simulink model "SSR_IFFT"  (R2020a)
settings: Solver=VariableStepAuto  StartTime=0.0  StopTime=2E-9*N/SSR*8  RelTol=1e-3
PreLoadFcn:
  | N=1024;
  | SSR=4;
undefined symbols (not defined in the file): Low
libraries: xbsIndex_r4 x10, xrbsSSR_Library x5, dspbuff3 x1, xbsCopyrightNotice_r4 x1, dspxfrm3 x1, dspswit3 x1
settings Model: Creator=admin  LastModifiedBy=viswanad
settings DataIOCC: ReturnWorkspaceOutputs=off
settings DebuggingCC: ArithmeticOperatorsInVariantConditions=warning
settings SFSimCC: SimUseLocalCustomCode=off  CustomCodeUndefinedFunction=UseInterfaceOnly
settings RTWCC: RTWUseLocalCustomCode=off
settings CodeAppCC: StateflowObjectComments=on

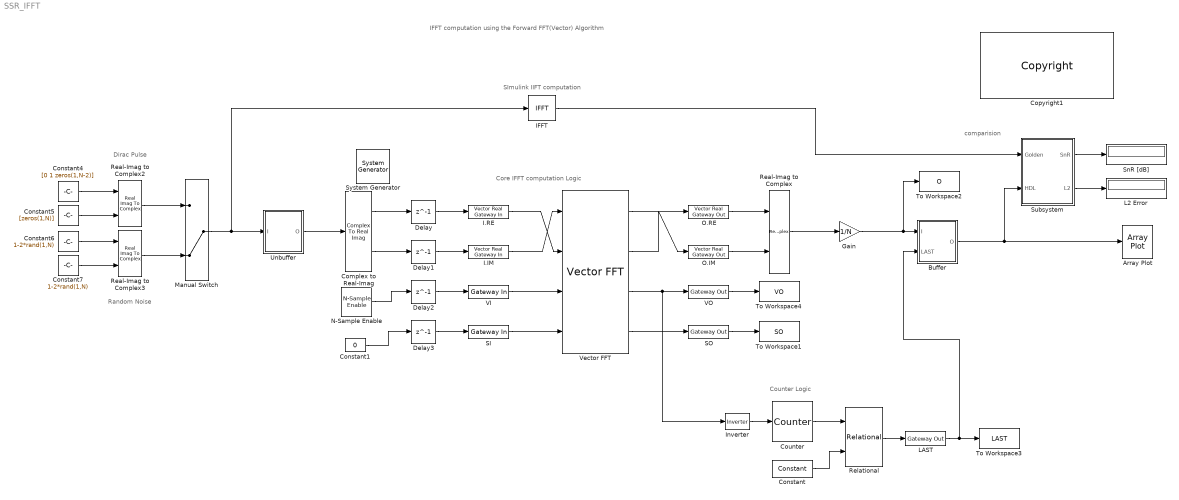
== system SSR_IFFT ==
  note: comparision
  note: Counter Logic
  note: SImulink IIFT computation
  note: Core IFFT computation Logic
  note: Dirac Pulse
  note: Random Noise
  note: IFFT computation using the Forward FFT(Vector)
      | Algorithm
  " System Generator" : xbsIndex_r4/ System Generator  Tag=genX  xilinxfamily=kintex7  part=xc7k325t  speed=-3  package=fbg676  synthesis_tool=Vivado  clock_wrapper=Clock Enables  directory=./netlist  proj_type=Vivado  Synth_file=Vivado Synthesis Defaults  Impl_file=Vivado Implementation Defaults  testbench=off  simulink_period=2E-09  sysclk_period=2  dcm_input_clock_period=10  incr_netlist=off  trim_vbits=Everywhere in SubSystem  dbl_ovrd=According to Block Masks  core_generation=According to Block Masks  run_coregen=off  deprecated_control=off  eval_field=0  block_type=sysgen
  Array Plot : ArrayPlot
  Buffer : Subsystem
  Complex to Real-Imag : ComplexToRealImag
  Constant : xbsIndex_r4/Constant  const=N/SSR-1  gui_display_data_type=Fixed-point  arith_type=Unsigned  n_bits=log2(N/SSR)  bin_pt=0  preci_type=Single  exp_width=8  frac_width=24  explicit_period=off  period=1  equ=P=C  opselect=C  inp2=PCIN>>17  opr=+  inp1=P  carry=CIN  dbl_ovrd=off  block_type=constant
  Constant1 : Constant  Value=0  SampleTime=-1
  Constant4 : Constant  Value=[0 1 zeros(1,N-2)]  SampleTime=-1
  Constant5 : Constant  Value=[zeros(1,N)]  SampleTime=-1
  Constant6 : Constant  Value=1-2*rand(1,N)  SampleTime=-1
  Constant7 : Constant  Value=1-2*rand(1,N)  SampleTime=-1
  Copyright1 : xbsCopyrightNotice_r4/Copyright  copyrighttext="Copyright (c) 2021  by  Xilinx, Inc. All rights reserved.<br><br>This file contains proprietary, confidential information of Xilinx, Inc., is distributed under license from Xilinx, Inc., and may be used, copied and/or disclosed only pursuant to the terms of a valid license agreement with Xilinx, Inc. Xilinx hereby grants you a license to use this file solely for design, simulation, implementation and creation of design files limited to Xilinx devices or technologies. Use with non-Xilinx devices or technologies is expressly prohibited and immediately terminates your license unless covered by a separate agreement.<br><br>Xilinx is providing this design, code, or information \"as-is\" solely for use in developing programs and solutions for Xilinx devices, with no obligation on the part of Xilinx to provide support. By providing this design, code, or information as one possible implementation of this feature, application or standard, Xilinx is making no representation that this implementation is free from any claims of infringement. You are responsible for obtaining any rights you may require for your implementation. Xilinx expressly disclaims any warranty whatsoever with respect to the adequacy of the implementation, including but not limited to any warranties or representations that this implementation is free from claims of infringement, implied warranties of merchantability or fitness for a particular purpose.<br><br>Xilinx products are not intended for use in life support appliances, devices, or systems. Use in such applications is expressly prohibited.<br><br>Any modifications that are made to the Source Code are done at the user's sole risk and will be unsupported.<br><br>This copyright and support notice must be retained as part of this text at all times. (c) Copyright 1995-2021 Xilinx, Inc. All rights reserved."  block_type=copyright
  Counter : xbsIndex_r4/Counter  cnt_type=Free Running  cnt_to=Inf  operation=Up  start_count=0  cnt_by_val=1  arith_type=Unsigned  n_bits=log2(N/SSR)  bin_pt=0  load_pin=off  rst=on  en=off  explicit_period=on  period=2E-9  use_behavioral_HDL=off  implementation=Fabric  dbl_ovrd=off  block_type=counter
  Delay{,1..3} (4 alike) : Delay  DelayLength=1
  Gain : Gain  Gain=1/N
  I.IM : xrbsSSR_Library/Vector Real Gateway In  gui_display_data_type=Fixed-point  arith_type="Signed  (2's comp)"  n_bits=18  bin_pt=16  preci_type=Single  exp_width=8  frac_width=24  quantization="Round  (unbiased: +/- Inf)"  overflow=Saturate  period=2E-9  sg_ssr=SSR  sg_ssr_prev=4  UseAsADC=off  ADCChannel='1'  interface=None  interface_prev=1  automatic_assignment=off  address_offset=hex2dec('00')  intf_name=''  intf_description=''  default_value=0  timing_constraint=None  locs_specified=off  LOCs={}  io_standard={}  hdl_port=on  dbl_ovrd=off  block_type=realgatewayin_ssr
      settings: SourceProductName=Xilinx SSR Blockset  infoedit=The Vector Real Gateway in block converts Vector inputs of type Simulink integer, single, double and fixed-point to Xilinx fixed-point or floating-point data type.<br><br>Hardware notes: In hardware these blocks become top level input ports.
  I.RE : xrbsSSR_Library/Vector Real Gateway In  gui_display_data_type=Fixed-point  arith_type="Signed  (2's comp)"  n_bits=18  bin_pt=16  preci_type=Single  exp_width=8  frac_width=24  quantization="Round  (unbiased: +/- Inf)"  overflow=Saturate  period=2E-9  sg_ssr=SSR  sg_ssr_prev=4  UseAsADC=off  ADCChannel='1'  interface=None  interface_prev=1  automatic_assignment=off  address_offset=hex2dec('00')  intf_name=''  intf_description=''  default_value=0  timing_constraint=None  locs_specified=off  LOCs={}  io_standard={}  hdl_port=on  dbl_ovrd=off  block_type=realgatewayin_ssr
      settings: SourceProductName=Xilinx SSR Blockset  infoedit=The Vector Real Gateway in block converts Vector inputs of type Simulink integer, single, double and fixed-point to Xilinx fixed-point or floating-point data type.<br><br>Hardware notes: In hardware these blocks become top level input ports.
  IFFT : dspxfrm3/IFFT  FFTImplementation=FFTW  CompMethod=Table lookup  TableOpt=NEW  TableOptActive=Speed  BitRevOrder=off  cs_in=off  Normalize=on  InheritFFTLength=on  FFTLength=64  WrapInput=on  mode=Complex  outSamplingMode=Sample based  roundingMode=Floor  overflowMode=off  firstCoeffDataTypeStr=Inherit: Same word length as input  firstCoeffLastDataTypeStr=Inherit: Same word length as input  outputMin=[]  outputMax=[]
  Inverter : xbsIndex_r4/Inverter  en=off  latency=0  dbl_ovrd=off  block_type=inv
  L2 Error : Display
  LAST : xbsIndex_r4/Gateway Out  inherit_from_input=off  hdl_port=on  rows=1  columns=1  UseAsDAC=off  DACChannel='1'  interface=None  automatic_assignment=on  address_offset=hex2dec('00')  intf_name=''  intf_description=''  timing_constraint=None  locs_specified=off  LOCs={}  io_standard={}  block_type=gatewayout
  Manual Switch : ManualSwitch  CurrentSetting=0
  N-Sample Enable : dspswit3/N-Sample Enable  N=N/SSR  ActiveLevel=Low (0)  reset=off  TriggerType=Rising edge  Ts=-1  DataType=Logical
      settings: SourceProductBaseCode=DS
  O.IM : xrbsSSR_Library/Vector Real Gateway Out  inherit_from_input=off  hdl_port=on  rows=1  columns=1  UseAsDAC=off  DACChannel='1'  interface=None  automatic_assignment=on  address_offset=hex2dec('00')  intf_name=''  intf_description=''  timing_constraint=None  locs_specified=off  LOCs={}  io_standard={}  block_type=realgatewayout_ssr  sg_ssr=SSR  sg_ssr_prev=4  sg_ssr_name=vect_real_gwayout
      settings: SourceProductName=Xilinx SSR Blockset  infoedit=The Vector Real Gateway out block converts Xilinx fixed-point or floating-point type vector inputs into vector ouputs of type Simulink integer, single, double, or fixed-point.<br><br>Hardware notes: In hardware these blocks become top level output ports or are discarded, depending on how they are configured.
  O.RE : xrbsSSR_Library/Vector Real Gateway Out  inherit_from_input=off  hdl_port=on  rows=1  columns=1  UseAsDAC=off  DACChannel='1'  interface=None  automatic_assignment=on  address_offset=hex2dec('00')  intf_name=''  intf_description=''  timing_constraint=None  locs_specified=off  LOCs={}  io_standard={}  block_type=realgatewayout_ssr  sg_ssr=SSR  sg_ssr_prev=4  sg_ssr_name=vect_real_gwayout
      settings: SourceProductName=Xilinx SSR Blockset  infoedit=The Vector Real Gateway out block converts Xilinx fixed-point or floating-point type vector inputs into vector ouputs of type Simulink integer, single, double, or fixed-point.<br><br>Hardware notes: In hardware these blocks become top level output ports or are discarded, depending on how they are configured.
  Real-Imag to Complex : RealImagToComplex
  Real-Imag to Complex2 : RealImagToComplex
  Real-Imag to Complex3 : RealImagToComplex
  Relational : xbsIndex_r4/Relational  mode=a=b  op_type=Bool  en=off  latency=1  dbl_ovrd=off  block_type=relational
  SI : xbsIndex_r4/Gateway In  gui_display_data_type=Fixed-point  arith_type=Unsigned  n_bits=log2(N)  bin_pt=0  preci_type=Single  exp_width=8  frac_width=24  rows=1  columns=1  quantization="Round  (unbiased: +/- Inf)"  overflow=Saturate  period=2E-9  UseAsADC=off  ADCChannel='1'  interface=None  automatic_assignment=on  address_offset=hex2dec('00')  intf_name=''  intf_description=''  default_value=0  timing_constraint=None  locs_specified=off  LOCs={}  io_standard={}  inherit_from_input=off  hdl_port=on  dbl_ovrd=off  block_type=gatewayin
  SO : xbsIndex_r4/Gateway Out  inherit_from_input=off  hdl_port=on  rows=1  columns=1  UseAsDAC=off  DACChannel='1'  interface=None  automatic_assignment=on  address_offset=hex2dec('00')  intf_name=''  intf_description=''  timing_constraint=None  locs_specified=off  LOCs={}  io_standard={}  block_type=gatewayout
  SnR [dB] : Display
  Subsystem : Subsystem
  To Workspace1 : ToWorkspace  VariableName=SO  SampleTime=-1
  To Workspace2 : ToWorkspace  VariableName=O  SampleTime=-1
  To Workspace3 : ToWorkspace  VariableName=LAST  SampleTime=-1
  To Workspace4 : ToWorkspace  VariableName=VO  SampleTime=-1
  Unbuffer : Subsystem
  VI : xbsIndex_r4/Gateway In  gui_display_data_type=Boolean  arith_type=Boolean  n_bits=16  bin_pt=14  preci_type=Single  exp_width=8  frac_width=24  rows=1  columns=1  quantization="Round  (unbiased: +/- Inf)"  overflow=Saturate  period=2E-9  UseAsADC=off  ADCChannel='1'  interface=None  automatic_assignment=on  address_offset=hex2dec('00')  intf_name=''  intf_description=''  default_value=0  timing_constraint=None  locs_specified=off  LOCs={}  io_standard={}  inherit_from_input=off  hdl_port=on  dbl_ovrd=off  block_type=gatewayin
  VO : xbsIndex_r4/Gateway Out  inherit_from_input=off  hdl_port=on  rows=1  columns=1  UseAsDAC=off  DACChannel='1'  interface=None  automatic_assignment=on  address_offset=hex2dec('00')  intf_name=''  intf_description=''  timing_constraint=None  locs_specified=off  LOCs={}  io_standard={}  block_type=gatewayout
  Vector FFT : xrbsSSR_Library/Vector FFT  sg_ssr=SSR  N=N  W_high=1  W_low=-17  n_bits=26  bin_pt=16  bram_threshold=258  block_type=fft_ssr  sg_ssr_prev=4
      settings: SourceProductName=Xilinx SSR Blockset
  wires:
  VI/1 -> Vector FFT/3
  Vector FFT/3 -> Inverter/1, VO/1
  SI/1 -> Vector FFT/4
  Vector FFT/4 -> SO/1
  O.RE/1 -> Real-Imag to Complex/1
  O.IM/1 -> Real-Imag to Complex/2
  SO/1 -> To Workspace1/1
  Constant1/1 -> Delay3/1
  Complex to Real-Imag/2 -> Delay1/1
  N-Sample Enable/1 -> Delay2/1
  Inverter/1 -> Counter/1
  Counter/1 -> Relational/1
  Constant/1 -> Relational/2
  Relational/1 -> LAST/1
  VO/1 -> To Workspace4/1
  Real-Imag to Complex2/1 -> Manual Switch/1
  Constant4/1 -> Real-Imag to Complex2/1
  Constant5/1 -> Real-Imag to Complex2/2
  Constant7/1 -> Real-Imag to Complex3/2
  Constant6/1 -> Real-Imag to Complex3/1
  Real-Imag to Complex3/1 -> Manual Switch/2
  Manual Switch/1 -> IFFT/1, Unbuffer/1(I)
  Buffer/1(O) -> Array Plot/1, Subsystem/2(HDL)
  Real-Imag to Complex/1 -> Gain/1
  LAST/1 -> Buffer/2(LAST), To Workspace3/1
  Subsystem/1(SnR) -> SnR [dB]/1
  Subsystem/2(L2) -> L2 Error/1
  Complex to Real-Imag/1 -> Delay/1
  Unbuffer/1(O) -> Complex to Real-Imag/1
  Delay/1 -> I.RE/1
  Delay1/1 -> I.IM/1
  Delay2/1 -> VI/1
  Delay3/1 -> SI/1
  I.IM/1 -> Vector FFT/1
  I.RE/1 -> Vector FFT/2
  Vector FFT/1 -> O.IM/1
  Vector FFT/2 -> O.RE/1
  IFFT/1 -> Subsystem/1(Golden)
  Gain/1 -> To Workspace2/1, Buffer/1(I)

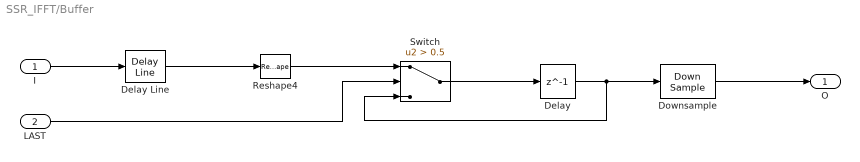
== system SSR_IFFT/Buffer ==
  I : Inport
  LAST : Inport  Port=2
  Delay : Delay  DelayLength=1
  Delay Line : dspbuff3/Delay Line  siz=N  ic=0  directfeed=off  enable_output=off  hold_output=off  OutputFrames=off
      settings: SourceProductBaseCode=DS
  Downsample : DownSample  N=N/SSR  RateOptions=Allow multirate processing
  Reshape4 : Reshape  OutputDimensions=[256,4]
  Switch : Switch  Criteria=u2 > Threshold  Threshold=0.5
  O : Outport  VectorParamsAs1DForOutWhenUnconnected=off
  wires:
  Switch/1 -> Delay/1
  I/1 -> Delay Line/1
  Downsample/1 -> O/1
  Delay/1 -> Switch/3, Downsample/1
  Delay Line/1 -> Reshape4/1
  Reshape4/1 -> Switch/1
  LAST/1 -> Switch/2

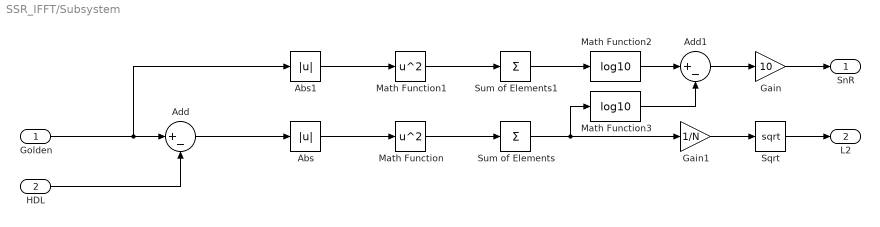
== system SSR_IFFT/Subsystem ==
  Golden : Inport
  HDL : Inport  Port=2
  Abs : Abs
  Abs1 : Abs
  Add : Sum  Inputs=|+-
  Add1 : Sum  Inputs=|+-
  Gain : Gain  Gain=10
  Gain1 : Gain  Gain=1/N
  Math Function : Math  Operator=square  SignedPower=on  SaturateOnIntegerOverflow=on
  Math Function1 : Math  Operator=square  SignedPower=on  SaturateOnIntegerOverflow=on
  Math Function2 : Math  Operator=log10  SignedPower=on  SaturateOnIntegerOverflow=on
  Math Function3 : Math  Operator=log10  SignedPower=on  SaturateOnIntegerOverflow=on
  Sqrt : Sqrt  SaturateOnIntegerOverflow=on
  Sum of Elements : Sum  Inputs=+
  Sum of Elements1 : Sum  Inputs=+
  SnR : Outport  VectorParamsAs1DForOutWhenUnconnected=off
  L2 : Outport  Port=2  VectorParamsAs1DForOutWhenUnconnected=off
  wires:
  Gain/1 -> SnR/1
  Add1/1 -> Gain/1
  Math Function3/1 -> Add1/2
  Math Function1/1 -> Sum of Elements1/1
  Sum of Elements1/1 -> Math Function2/1
  Abs1/1 -> Math Function1/1
  Math Function/1 -> Sum of Elements/1
  Sum of Elements/1 -> Math Function3/1, Gain1/1
  Golden/1 -> Abs1/1, Add/1
  Math Function2/1 -> Add1/1
  Abs/1 -> Math Function/1
  Add/1 -> Abs/1
  HDL/1 -> Add/2
  Sqrt/1 -> L2/1
  Gain1/1 -> Sqrt/1

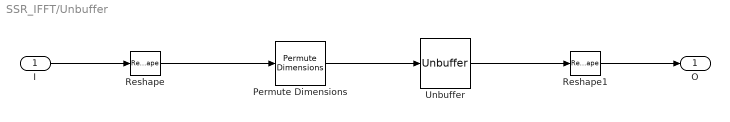
== system SSR_IFFT/Unbuffer ==
  I : Inport
  Permute Dimensions : PermuteDimensions
  Reshape : Reshape  OutputDimensionality=Customize  OutputDimensions=[SSR,N/SSR]
  Reshape1 : Reshape  OutputDimensions=[256,4]
  Unbuffer : Unbuffer
  O : Outport  VectorParamsAs1DForOutWhenUnconnected=off
  wires:
  Unbuffer/1 -> Reshape1/1
  Permute Dimensions/1 -> Unbuffer/1
  Reshape/1 -> Permute Dimensions/1
  Reshape1/1 -> O/1
  I/1 -> Reshape/1
